simulink model "controller"  (R2024b)
settings: Solver=VariableStepAuto  StartTime=0.0  StopTime=10.0  FixedStep=T  RelTol=1e-3
settings Model: DataDictionary=wrapper2.sldd  Creator=maciej  LastModifiedBy=maciej

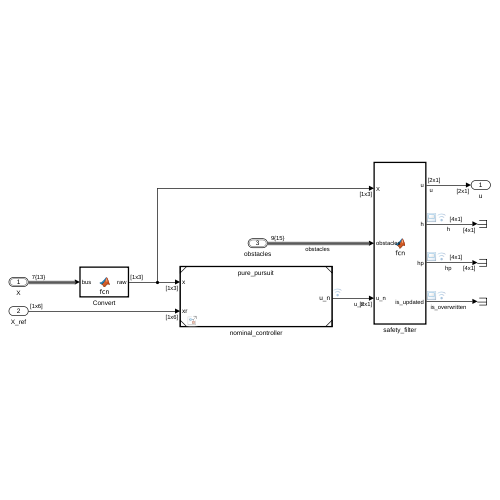
[thumbnail: Simulink's stored preview of the top-level diagram]
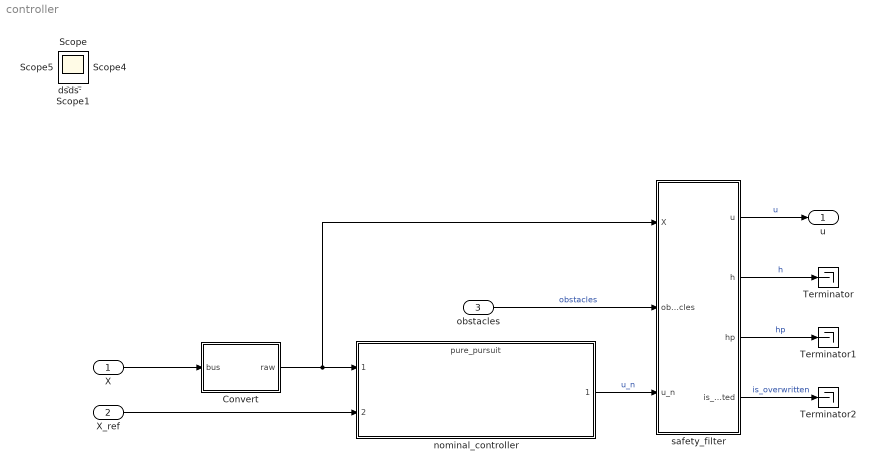
== system controller ==
  X : Inport  OutDataTypeStr=Bus: EgoVehicle  PortDimensions=1
  X_ref : Inport  Port=2  OutDataTypeStr=double  PortDimensions=[1, 6]
  obstacles : Inport  Port=3  OutDataTypeStr=Bus: Actors
  Convert : MATLAB Function  TreatAsAtomicUnit=on
  Terminator : Terminator
  Terminator1 : Terminator
  Terminator2 : Terminator
  nominal_controller : ModelReference  ModelNameDialog=pure_pursuit.slx  SimulationMode=Normal  ModelReferenceVersion=1.292
  safety_filter : MATLAB Function  TreatAsAtomicUnit=on
  u : Outport
  CBF : Scope
  Scope{,1,4..5} (4 alike) : Scope
  dsds : Scope
  wires:
  X/1 -> Convert/1(bus)
  Convert/1(raw) -> safety_filter/1(X), nominal_controller/1
  obstacles/1 -> safety_filter/2(obstacles)  "obstacles"
  safety_filter/2(h) -> Terminator/1  "h"
  safety_filter/3(hp) -> Terminator1/1  "hp"
  safety_filter/4(is_updated) -> Terminator2/1  "is_overwritten"
  nominal_controller/1 -> safety_filter/3(u_n)  "u_n"
  X_ref/1 -> nominal_controller/2
  safety_filter/1(u) -> u/1  "u"

== matlab function controller/Convert ==
  data: bus input Bus: EgoVehicle; raw output size=[1 3]
function raw = fcn(bus)
    raw = [ ...
        bus.Position(1), ...
        bus.Position(2), ...
        deg2rad(bus.Yaw) ...
    ];
end

== matlab function controller/safety_filter ==
  data: X input; u output; h output; obstacles input Bus: Actors; u_n input; hp output; is_updated output
function [u, h, hp, is_updated] = fcn(X, obstacles, u_n)
    x = X(1);
    y = X(2);
    theta = X(3);

    xo1 = 5;%obstacles.Actors(1).Position(1);
    yo1 = 0;%obstacles.Actors(1).Position(2);
    
    h1 = ((x - xo1)^2 +(y - yo1)^2 +  theta^2) - 1.5;
    dh1 = [2*x - 2*xo1, 2*y - 2*yo1, 2* theta];

    xo2 = 20;%obstacles.Actors(1).Position(1);
    yo2 = 0.5;%obstacles.Actors(1).Position(2);

    h2 = ((x - xo2)^2 +(y - yo2)^2 +  theta^2) - 1.5;
    dh2 = [2*x - 2*xo2, 2*y - 2*yo2, 2* theta];

    xo3 = 30;%obstacles.Actors(1).Position(1);
    yo3 = -1;%obstacles.Actors(1).Position(2);

    h3 = ((x - xo3)^2 +(y - yo3)^2 +  theta^2) - 1.5;
    dh3 = [2*x - 2*xo3, 2*y - 2*yo3, 2* theta];

    xo4 = 29;%obstacles.Actors(1).Position(1);
    yo4 = 2;%obstacles.Actors(1).Position(2);

    h4 = ((x - xo4)^2 +(y - yo4)^2 +  theta^2) - 1.5;
    dh4 = [2*x - 2*xo4, 2*y - 2*yo4, 2* theta];
    
    f = [0;0;0];
    g = [cos(theta) 0; sin(theta) 0; 0 1];
    
    q = @(ub)norm(ub-u_n)^2;
    x0 = u_n;
    A1 = -dh1*g;
    b1 = dh1*f + 2.5*h1;
    A2 = -dh2*g;
    b2 = dh2*f + 2.5*h2;
    A3 = -dh3*g;
    b3 = dh3*f + 2.5*h3;
    A4 = -dh4*g;
    b4 = dh4*f + 2.5*h4;
    options = optimoptions('fmincon', 'Algorithm', 'sqp', 'Display', 'off');
    u = fmincon(q, x0, [A1;A2;A3;A4], [b1;b2;b3;b4], [], [], [0.05 -1000], [], [], options);

    h = [h1; h2; h3; h4];
    hp = [dh1*f + dh1*g*u; dh2*f + dh2*g*u; dh3*f + dh3*g*u; dh4*f + dh4*g*u];

    is_updated = abs(norm(u_n) - norm(u)) > 0.01;
end
